simulink model "delta_coils"  (R2021a)
settings: Solver=VariableStepAuto  StartTime=0.0  StopTime=0.1  RelTol=1e-3
values from neighbouring files (symbols this model uses):
  carrier_B = 0    [param.m]    (also in parametic_sweep.m = [])
  carrier_C = 0    [param.m]    (also in parametic_sweep.m = [])
  fo = 100    [param.m]    (also in parametic_sweep.m)
  fsw = 50e3    (= 50000)    [param.m]    (also in parametic_sweep.m)
  ma = 0.8    [param.m]    (also in parametic_sweep.m = 0.5)
undefined symbols (not defined in the file or in its folder): MagA_f, MagA_l, MagB_f, MagB_l, MagC_f, MagC_l, PhaseA_f, PhaseA_h, PhaseA_l, PhaseB_f, PhaseB_h, PhaseB_l, PhaseC_f, PhaseC_h, PhaseC_l
libraries: spsACVoltageSourceLib x9, spsControlledVoltageSourceLib x3, spsCurrentMeasurementLib x3, spsSeriesRLCBranchLib x3, spsVoltageMeasurementLib x2, spspowerguiLib x1
settings Model: Creator=enes_  LastModifiedBy=enes_
settings DataIOCC: ReturnWorkspaceOutputs=off

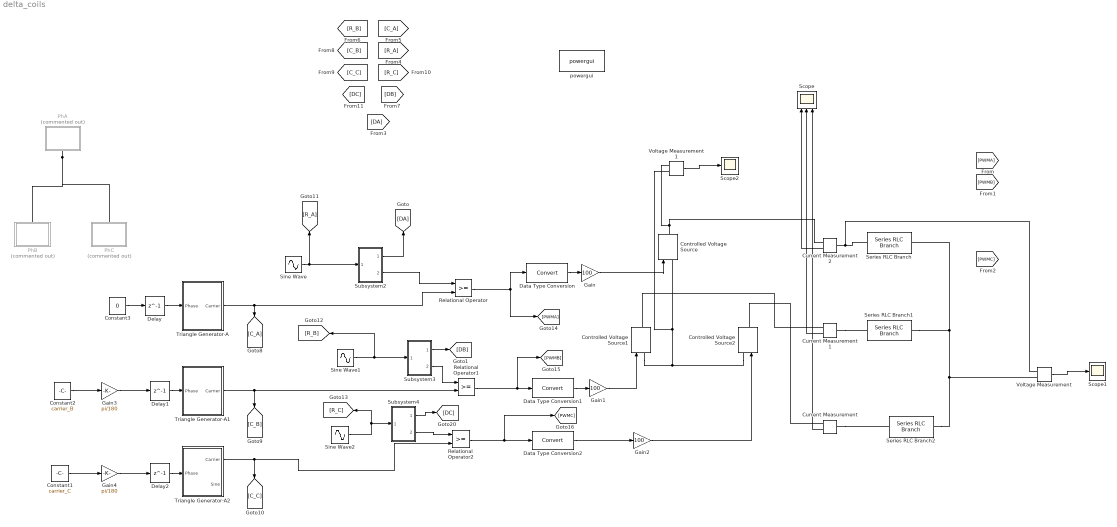
== system delta_coils ==
  Constant1 : Constant  Value=carrier_C
  Constant2 : Constant  Value=carrier_B
  Constant3 : Constant  Value=0
  Controlled Voltage Source : spsControlledVoltageSourceLib/Controlled Voltage Source  Initialize=on  Source_Type=AC  Amplitude=0  Phase=0  Frequency=0  Measurements=None
  Controlled Voltage Source1 : spsControlledVoltageSourceLib/Controlled Voltage Source  Initialize=on  Source_Type=AC  Amplitude=0  Phase=0  Frequency=0  Measurements=None
  Controlled Voltage Source2 : spsControlledVoltageSourceLib/Controlled Voltage Source  Initialize=on  Source_Type=AC  Amplitude=0  Phase=0  Frequency=0  Measurements=None
  Current Measurement : spsCurrentMeasurementLib/Current Measurement  PhasorSimulation=off  OutputType=Complex  PSBequivalent=0
  Current Measurement1 : spsCurrentMeasurementLib/Current Measurement  PhasorSimulation=off  OutputType=Complex  PSBequivalent=0
  Current Measurement2 : spsCurrentMeasurementLib/Current Measurement  PhasorSimulation=off  OutputType=Complex  PSBequivalent=0
  Data Type Conversion : DataTypeConversion
  Data Type Conversion1 : DataTypeConversion
  Data Type Conversion2 : DataTypeConversion
  Delay : Delay  DelayLength=1
  Delay1 : Delay  DelayLength=1
  Delay2 : Delay  DelayLength=1
  Gain : Gain  Gain=100
  Gain1 : Gain  Gain=100
  Gain2 : Gain  Gain=100
  Gain3 : Gain  Gain=pi/180
  Gain4 : Gain  Gain=pi/180
  PhA : Subsystem  Commented=on
  PhB : Subsystem  Commented=on
  PhC : Subsystem  Commented=on
  Relational Operator : RelationalOperator  OutDataTypeStr=boolean  RndMeth=Simplest
  Relational Operator1 : RelationalOperator  OutDataTypeStr=boolean  RndMeth=Simplest
  Relational Operator2 : RelationalOperator  OutDataTypeStr=boolean  RndMeth=Simplest
  Scope : Scope  NumInputPorts=3
  Scope1 : Scope
  Scope2 : Scope
  Series RLC Branch : spsSeriesRLCBranchLib/Series RLC Branch  LConnTagsString=__new0  RConnTagsString=__new0  BranchType=R  Resistance=1  Inductance=1e-3  SetiL0=off  InitialCurrent=0  Capacitance=1e-6  Setx0=off  InitialVoltage=0  Measurements=None
  Series RLC Branch1 : spsSeriesRLCBranchLib/Series RLC Branch  LConnTagsString=__new0  RConnTagsString=__new0  BranchType=R  Resistance=1  Inductance=1e-3  SetiL0=off  InitialCurrent=0  Capacitance=1e-6  Setx0=off  InitialVoltage=0  Measurements=None
  Series RLC Branch2 : spsSeriesRLCBranchLib/Series RLC Branch  LConnTagsString=__new0  RConnTagsString=__new0  BranchType=R  Resistance=1  Inductance=1e-3  SetiL0=off  InitialCurrent=0  Capacitance=1e-6  Setx0=off  InitialVoltage=0  Measurements=None
  Sine Wave : Sin  Amplitude=ma  Frequency=2*pi*fo  SampleTime=0
  Sine Wave1 : Sin  Amplitude=ma  Frequency=2*pi*fo  Phase=2*pi/3  SampleTime=0
  Sine Wave2 : Sin  Amplitude=ma  Frequency=2*pi*fo  Phase=-2*pi/3  SampleTime=0
  Subsystem2 : Subsystem
  Subsystem3 : Subsystem
  Subsystem4 : Subsystem
  Triangle Generator-A : Subsystem
  Triangle Generator-A1 : Subsystem
  Triangle Generator-A2 : Subsystem
  Voltage Measurement : spsVoltageMeasurementLib/Voltage Measurement  PhasorSimulation=off  OutputType=Complex  PSBequivalent=0
  Voltage Measurement1 : spsVoltageMeasurementLib/Voltage Measurement  PhasorSimulation=off  OutputType=Complex  PSBequivalent=0
  powergui : spspowerguiLib/powergui  Priority=1  SimulationMode=Discrete  SampleTime=1e-7  frequency=60  Iterations=50  frequencyindice=0  Pbase=100e6  ErrMax=1e-4  UnitsV=kV  UnitsW=MW  buscounter=0  FunctionMessages=off  echomessages=off  EnableUseOfTLC=off  CurrentSourceSwitches=off  DisableSnubberDevices=off  DisableRonSwitches=off  DisableVfSwitches=off  DisplayEquations=off  AutomaticDiscreteSolvers=off  SolverType=Tustin/Backward Euler (TBE)  Interpol=off  ExternalGateDelay=off  methode=off  Ts=100  x0status=blocks  SPID=on  SwTol=0  HookPort=off  NonlinearTolerance=1e-4  nMaxIteration=100  ContinueOnMaxIteration=off  RestoreLinks=warning  ResistiveCurrentMeasurement=off  Frange=[0:2:500]  Ylog=off  Xlog=on  ShowGrid=off  save=off  variable=ZData  structure=0  ZoomFFT=off  StartTime=0.0  cycles=1  DisplayStyle=1  fundamental=60  FreqAxis=off  MaxFrequency=1000  frequencyindicesteady=1  RmsSteady=1  display=off
  wires:
  Sine Wave2/1 -> [R_C], Subsystem4/1(In1)
  Subsystem4/1(Out1) -> [DC]
  Subsystem4/2(Out2) -> Relational Operator2/1
  Subsystem3/1(Out1) -> [DB]
  Constant3/1 -> Delay/1
  Triangle Generator-A/1(Carrier) -> Relational Operator/2, [C_A]
  Triangle Generator-A1/1(Carrier) -> Relational Operator1/2, [C_B]
  Delay/1 -> Triangle Generator-A/1(Phase)
  Subsystem2/1(Out1) -> [DA]
  Sine Wave1/1 -> [R_B], Subsystem3/1(In1)
  Sine Wave/1 -> Subsystem2/1(In1), [R_A]
  Relational Operator/1 -> Data Type Conversion/1, [PWMA]
  Subsystem2/2(Out2) -> Relational Operator/1
  Relational Operator2/1 -> Data Type Conversion2/1, [PWMC]
  Subsystem3/2(Out2) -> Relational Operator1/1
  Delay2/1 -> Triangle Generator-A2/1(Phase)
  Delay1/1 -> Triangle Generator-A1/1(Phase)
  Relational Operator1/1 -> Data Type Conversion1/1, [PWMB]
  Triangle Generator-A2/1(Carrier) -> Relational Operator2/2, [C_C]
  Gain/1 -> Controlled Voltage Source/1
  Gain1/1 -> Controlled Voltage Source1/1
  Gain2/1 -> Controlled Voltage Source2/1
  Current Measurement2/1 -> Scope/1
  Current Measurement1/1 -> Scope/2
  Current Measurement/1 -> Scope/3
  Data Type Conversion/1 -> Gain/1
  Data Type Conversion1/1 -> Gain1/1
  Data Type Conversion2/1 -> Gain2/1
  Gain3/1 -> Delay1/1
  Constant2/1 -> Gain3/1
  Gain4/1 -> Delay2/1
  Constant1/1 -> Gain4/1
  Voltage Measurement/1 -> Scope1/1
  Voltage Measurement1/1 -> Scope2/1
  connections:
  PhA/LConn1 -- PhB/LConn1 -- PhC/LConn1
  Current Measurement2/LConn1 -- Series RLC Branch/LConn1 -- Voltage Measurement/LConn1
  Current Measurement/LConn1 -- Series RLC Branch2/LConn1
  Series RLC Branch2/RConn1 -- Voltage Measurement/LConn2 -- Series RLC Branch/RConn1 -- Series RLC Branch1/LConn1
  Controlled Voltage Source1/LConn1 -- Controlled Voltage Source2/LConn1 -- Controlled Voltage Source/LConn1 -- Voltage Measurement1/LConn2
  Current Measurement1/LConn1 -- Series RLC Branch1/RConn1
  Controlled Voltage Source/RConn1 -- Voltage Measurement1/LConn1 -- Current Measurement2/RConn1
  Current Measurement1/RConn1 -- Controlled Voltage Source1/RConn1
  Current Measurement/RConn1 -- Controlled Voltage Source2/RConn1

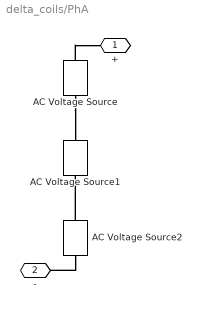
== system delta_coils/PhA ==
  AC Voltage Source : spsACVoltageSourceLib/AC Voltage Source  Amplitude=MagA_l  Phase=PhaseA_l  Frequency=fsw-2*fo  SampleTime=0  Measurements=None  BusType=swing  Pref=10e3  Qref=0  Qmin=-inf  Qmax=+inf
  AC Voltage Source1 : spsACVoltageSourceLib/AC Voltage Source  Amplitude=MagA_f  Phase=PhaseA_f  Frequency=fsw  SampleTime=0  Measurements=None  BusType=swing  Pref=10e3  Qref=0  Qmin=-inf  Qmax=+inf
  AC Voltage Source2 : spsACVoltageSourceLib/AC Voltage Source  Amplitude=MagA_l  Phase=PhaseA_h  Frequency=fsw+2*fo  SampleTime=0  Measurements=None  BusType=swing  Pref=10e3  Qref=0  Qmin=-inf  Qmax=+inf
  + : PMIOPort  Side=Right
  - : PMIOPort  Port=2  Side=Left
  connections:
  AC Voltage Source/LConn1 -- AC Voltage Source1/RConn1
  AC Voltage Source2/LConn1 -- -/RConn1
  AC Voltage Source/RConn1 -- +/RConn1
  AC Voltage Source2/RConn1 -- AC Voltage Source1/LConn1

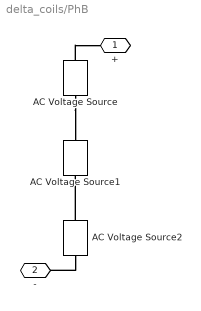
== system delta_coils/PhB ==
  AC Voltage Source : spsACVoltageSourceLib/AC Voltage Source  Amplitude=MagB_l  Phase=PhaseB_l  Frequency=fsw-2*fo  SampleTime=0  Measurements=None  BusType=swing  Pref=10e3  Qref=0  Qmin=-inf  Qmax=+inf
  AC Voltage Source1 : spsACVoltageSourceLib/AC Voltage Source  Amplitude=MagB_f  Phase=PhaseB_f  Frequency=fsw  SampleTime=0  Measurements=None  BusType=swing  Pref=10e3  Qref=0  Qmin=-inf  Qmax=+inf
  AC Voltage Source2 : spsACVoltageSourceLib/AC Voltage Source  Amplitude=MagB_l  Phase=PhaseB_h  Frequency=fsw+2*fo  SampleTime=0  Measurements=None  BusType=swing  Pref=10e3  Qref=0  Qmin=-inf  Qmax=+inf
  + : PMIOPort  Side=Right
  - : PMIOPort  Port=2  Side=Left
  connections:
  AC Voltage Source/LConn1 -- AC Voltage Source1/RConn1
  AC Voltage Source2/LConn1 -- -/RConn1
  AC Voltage Source/RConn1 -- +/RConn1
  AC Voltage Source2/RConn1 -- AC Voltage Source1/LConn1

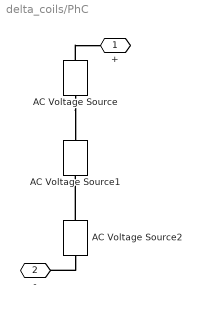
== system delta_coils/PhC ==
  AC Voltage Source : spsACVoltageSourceLib/AC Voltage Source  Amplitude=MagC_l  Phase=PhaseC_l  Frequency=fsw-2*fo  SampleTime=0  Measurements=None  BusType=swing  Pref=10e3  Qref=0  Qmin=-inf  Qmax=+inf
  AC Voltage Source1 : spsACVoltageSourceLib/AC Voltage Source  Amplitude=MagC_f  Phase=PhaseC_f  Frequency=fsw  SampleTime=0  Measurements=None  BusType=swing  Pref=10e3  Qref=0  Qmin=-inf  Qmax=+inf
  AC Voltage Source2 : spsACVoltageSourceLib/AC Voltage Source  Amplitude=MagC_l  Phase=PhaseC_h  Frequency=fsw+2*fo  SampleTime=0  Measurements=None  BusType=swing  Pref=10e3  Qref=0  Qmin=-inf  Qmax=+inf
  + : PMIOPort  Side=Right
  - : PMIOPort  Port=2  Side=Left
  connections:
  AC Voltage Source/LConn1 -- AC Voltage Source1/RConn1
  AC Voltage Source2/LConn1 -- -/RConn1
  AC Voltage Source/RConn1 -- +/RConn1
  AC Voltage Source2/RConn1 -- AC Voltage Source1/LConn1

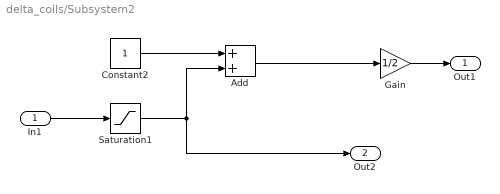
== system delta_coils/Subsystem2 ==
  In1 : Inport
  Add : Sum
  Constant2 : Constant
  Gain : Gain  Gain=1/2
  Saturation1 : Saturate  UpperLimit=1  LowerLimit=-1
  Out1 : Outport
  Out2 : Outport  Port=2
  wires:
  Constant2/1 -> Add/1
  Add/1 -> Gain/1
  Gain/1 -> Out1/1
  In1/1 -> Saturation1/1
  Saturation1/1 -> Out2/1, Add/2

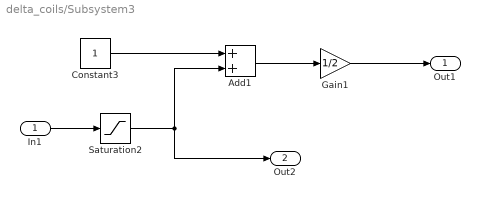
== system delta_coils/Subsystem3 ==
  In1 : Inport
  Add1 : Sum
  Constant3 : Constant
  Gain1 : Gain  Gain=1/2
  Saturation2 : Saturate  UpperLimit=1  LowerLimit=-1
  Out1 : Outport
  Out2 : Outport  Port=2
  wires:
  Saturation2/1 -> Out2/1, Add1/2
  In1/1 -> Saturation2/1
  Constant3/1 -> Add1/1
  Add1/1 -> Gain1/1
  Gain1/1 -> Out1/1

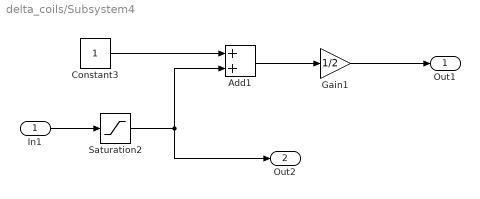
== system delta_coils/Subsystem4 ==
  In1 : Inport
  Add1 : Sum
  Constant3 : Constant
  Gain1 : Gain  Gain=1/2
  Saturation2 : Saturate  UpperLimit=1  LowerLimit=-1
  Out1 : Outport
  Out2 : Outport  Port=2
  wires:
  Saturation2/1 -> Out2/1, Add1/2
  In1/1 -> Saturation2/1
  Constant3/1 -> Add1/1
  Add1/1 -> Gain1/1
  Gain1/1 -> Out1/1

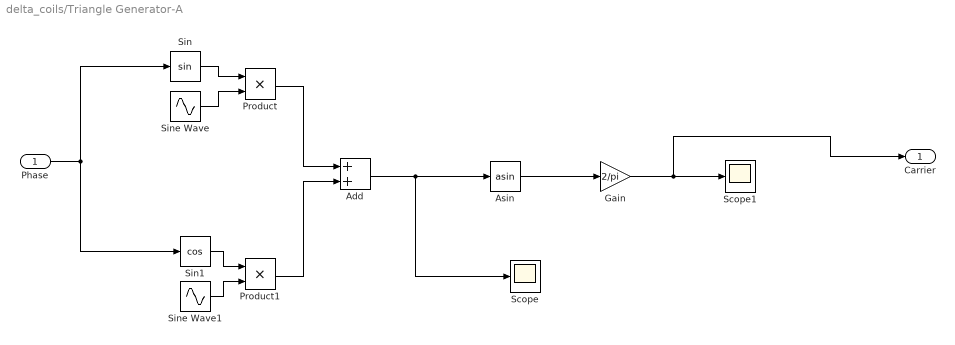
== system delta_coils/Triangle Generator-A ==
  Phase : Inport
  Add : Sum
  Asin : Trigonometry  Operator=asin
  Gain : Gain  Gain=2/pi
  Product : Product
  Product1 : Product
  Scope : Scope
  Scope1 : Scope
  Sin : Trigonometry
  Sin1 : Trigonometry  Operator=cos
  Sine Wave : Sin  Frequency=2*pi*fsw  SampleTime=0
  Sine Wave1 : Sin  Frequency=2*pi*fsw  Phase=-pi/2  SampleTime=0
  Carrier : Outport
  wires:
  Sin/1 -> Product/1
  Sine Wave/1 -> Product/2
  Phase/1 -> Sin1/1, Sin/1
  Product/1 -> Add/1
  Asin/1 -> Gain/1
  Gain/1 -> Carrier/1, Scope1/1
  Sine Wave1/1 -> Product1/2
  Product1/1 -> Add/2
  Add/1 -> Asin/1, Scope/1
  Sin1/1 -> Product1/1

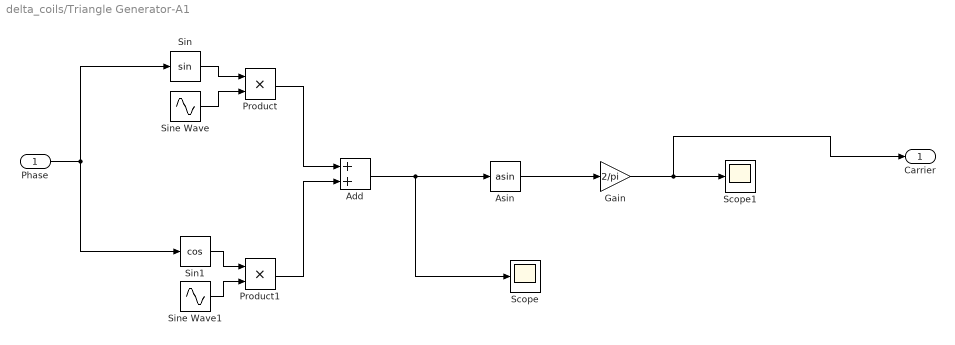
== system delta_coils/Triangle Generator-A1 ==
  Phase : Inport
  Add : Sum
  Asin : Trigonometry  Operator=asin
  Gain : Gain  Gain=2/pi
  Product : Product
  Product1 : Product
  Scope : Scope
  Scope1 : Scope
  Sin : Trigonometry
  Sin1 : Trigonometry  Operator=cos
  Sine Wave : Sin  Frequency=2*pi*fsw  SampleTime=0
  Sine Wave1 : Sin  Frequency=2*pi*fsw  Phase=-pi/2  SampleTime=0
  Carrier : Outport
  wires:
  Sin/1 -> Product/1
  Sine Wave/1 -> Product/2
  Phase/1 -> Sin1/1, Sin/1
  Product/1 -> Add/1
  Asin/1 -> Gain/1
  Gain/1 -> Carrier/1, Scope1/1
  Sine Wave1/1 -> Product1/2
  Product1/1 -> Add/2
  Add/1 -> Asin/1, Scope/1
  Sin1/1 -> Product1/1

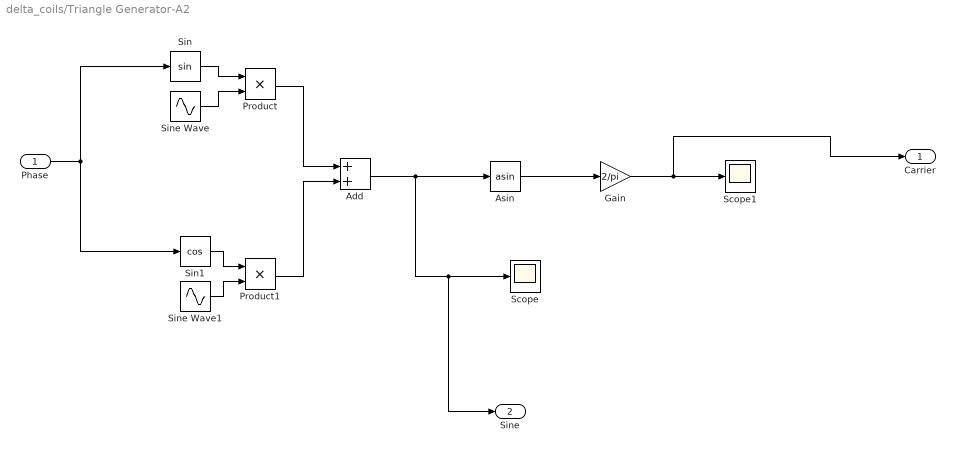
== system delta_coils/Triangle Generator-A2 ==
  Phase : Inport
  Add : Sum
  Asin : Trigonometry  Operator=asin
  Gain : Gain  Gain=2/pi
  Product : Product
  Product1 : Product
  Scope : Scope
  Scope1 : Scope
  Sin : Trigonometry
  Sin1 : Trigonometry  Operator=cos
  Sine Wave : Sin  Frequency=2*pi*fsw  SampleTime=0
  Sine Wave1 : Sin  Frequency=2*pi*fsw  Phase=-pi/2  SampleTime=0
  Carrier : Outport
  Sine : Outport  Port=2
  wires:
  Sin/1 -> Product/1
  Sine Wave/1 -> Product/2
  Phase/1 -> Sin1/1, Sin/1
  Product/1 -> Add/1
  Asin/1 -> Gain/1
  Gain/1 -> Carrier/1, Scope1/1
  Sine Wave1/1 -> Product1/2
  Product1/1 -> Add/2
  Add/1 -> Asin/1, Sine/1, Scope/1
  Sin1/1 -> Product1/1
